simulink model "cstr_mhe"  (R2014a)
settings: Solver=ode45  StartTime=0.0  StopTime=10  RelTol=1e-3
StartFcn:
  | clear all
  | close all
  | clc
StopFcn:
  | plot_reactor
  | clear all
libraries: simulink x4
settings Model: Creator=tsladeche  LastModifiedBy=John
settings DataIOCC: SignalLoggingSaveFormat=ModelDataLogs
settings OptimizationCC: ExpressionDepthLimit=2147483647
settings DebuggingCC: UnderspecifiedInitializationDetection=Classic  FcnCallInpInsideContextMsg=UseLocalSettings  StateNameClashWarn=warning
settings GRTTargetCC: CombineOutputUpdateFcns=off  GRTInterface=on

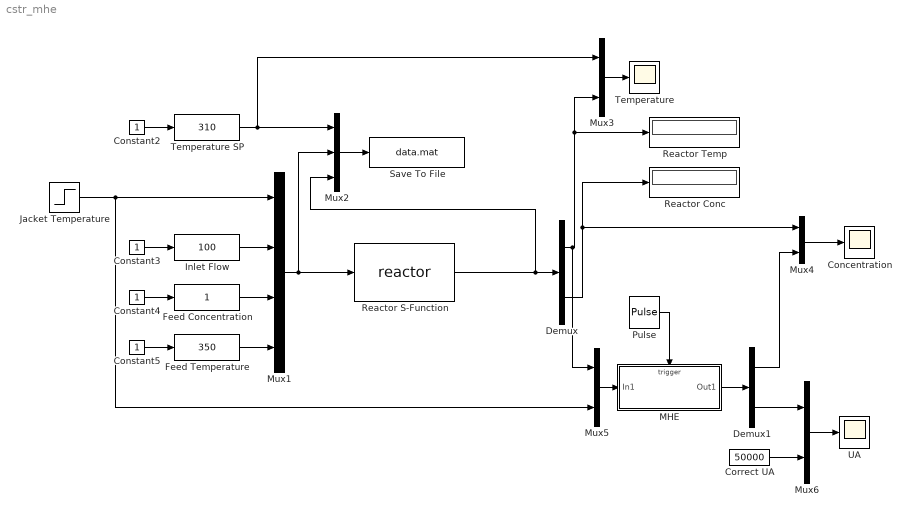
== system cstr_mhe ==
  Concentration : Scope
      settings: ShowLegends=on  YMin=0  YMax=1
  Constant{2..5} (4 alike) : Constant
  Correct UA : Constant  Value=50000
  Demux : Demux  Outputs=2
  Demux1 : Demux  Outputs=2
  Feed Concentration : simulink/Math Operations/Slider Gain  low=0  gain=1  high=1
  Feed Temperature : simulink/Math Operations/Slider Gain  low=300  gain=350  high=400
  Inlet Flow : simulink/Math Operations/Slider Gain  low=0  gain=100  high=200
  Jacket Temperature : Step  Before=280  After=300  SampleTime=0
  MHE : Subsystem  TreatAsAtomicUnit=on
  Mux1 : Mux
  Mux2 : Mux  Inputs=3
  Mux{3..6} (4 alike) : Mux  Inputs=2
  Pulse : DiscretePulseGenerator  PulseType=Time based  Period=0.1  PulseWidth=5
  Reactor Conc : Display
  Reactor S-Function : S-Function  FunctionName=reactor  EnableBusSupport=off
  Reactor Temp : Display
  Save To File : ToFile  Filename=data.mat  MatrixName=cstr  SampleTime=0.05
  Temperature : Scope
      settings: ShowLegends=on  TimeRange=10  YMin=285  YMax=400  MaxDataPoints=30000
  Temperature SP : simulink/Math Operations/Slider Gain  low=300  gain=310  high=400
  UA : Scope
      settings: ShowLegends=on  YMin=0  YMax=1  SaveName=ScopeData2
  wires:
  Reactor S-Function/1 -> Mux2/3, Demux/1
  Constant3/1 -> Inlet Flow/1
  Mux2/1 -> Save To File/1
  Mux1/1 -> Mux2/2, Reactor S-Function/1
  Inlet Flow/1 -> Mux1/2
  Constant2/1 -> Temperature SP/1
  Temperature SP/1 -> Mux3/1, Mux2/1
  Demux/2 -> Mux4/1, Reactor Conc/1
  Constant4/1 -> Feed Concentration/1
  Feed Concentration/1 -> Mux1/3
  Constant5/1 -> Feed Temperature/1
  Feed Temperature/1 -> Mux1/4
  Demux/1 -> Mux5/1, Mux3/2, Reactor Temp/1
  Mux3/1 -> Temperature/1
  Mux4/1 -> Concentration/1
  Pulse/1 -> MHE/Trigger
  Mux5/1 -> MHE/1(In1)
  Jacket Temperature/1 -> Mux1/1, Mux5/2
  MHE/1(Out1) -> Demux1/1
  Demux1/1 -> Mux4/2
  Demux1/2 -> Mux6/1
  Correct UA/1 -> Mux6/2
  Mux6/1 -> UA/1

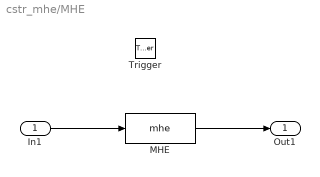
== system cstr_mhe/MHE ==
  In1 : Inport
  Trigger : TriggerPort
  MHE : MATLABFcn  MATLABFcn=mhe  OutputDimensions=2
  Out1 : Outport
  wires:
  In1/1 -> MHE/1
  MHE/1 -> Out1/1
